simulink model "diff_equiation"  (R2018b)
settings: Solver=VariableStepAuto  StartTime=0.0  StopTime=10.0  RelTol=1e-3
settings Model: Creator=Ismael  LastModifiedBy=Ismael

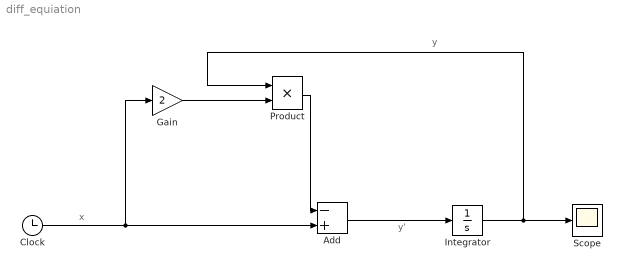
== system diff_equiation ==
  note: x
  note: y'
  note: y
  Add : Sum  Inputs=-+
  Clock : Clock
  Gain : Gain  Gain=2
  Integrator : Integrator  InitialCondition=1
  Product : Product
  Scope : Scope
  wires:
  Add/1 -> Integrator/1
  Product/1 -> Add/1
  Integrator/1 -> Product/1, Scope/1
  Clock/1 -> Gain/1, Add/2
  Gain/1 -> Product/2
